simulink model "GA_fuzzy_sim"  (R2023a)
settings: Solver=VariableStepAuto  StartTime=0.0  StopTime=5  RelTol=1e-3
InitFcn:
  | m0=0.8; m1=0.5; m2=0.3; L1=0.3; L2=0.2; l1=0.15; l2=0.1; I1=0.015; I2=0.004; g=9.8;
  | d1=(m0+m1+m2);
  | d2=(m1*l1+m2*L1);
  | d3=m1*l1^2+m2*L1^2+I1;
  | d4=m2*l2;
  | d5=m2*L1*l2;
  | d6=m2*l2^2+I2;
libraries: fuzblock x1
settings Model: Creator=luand  LastModifiedBy=luand
settings DataIOCC: ReturnWorkspaceOutputs=off

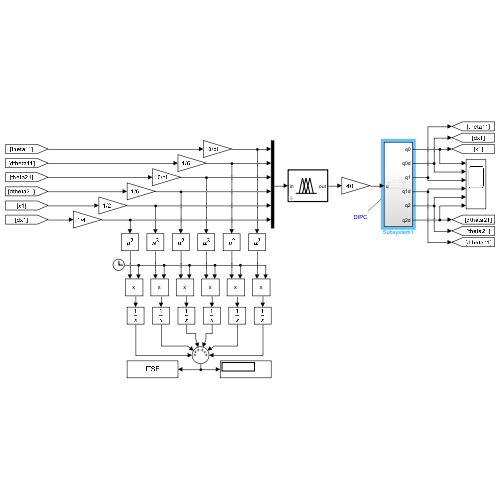
[thumbnail: Simulink's stored preview of the top-level diagram]
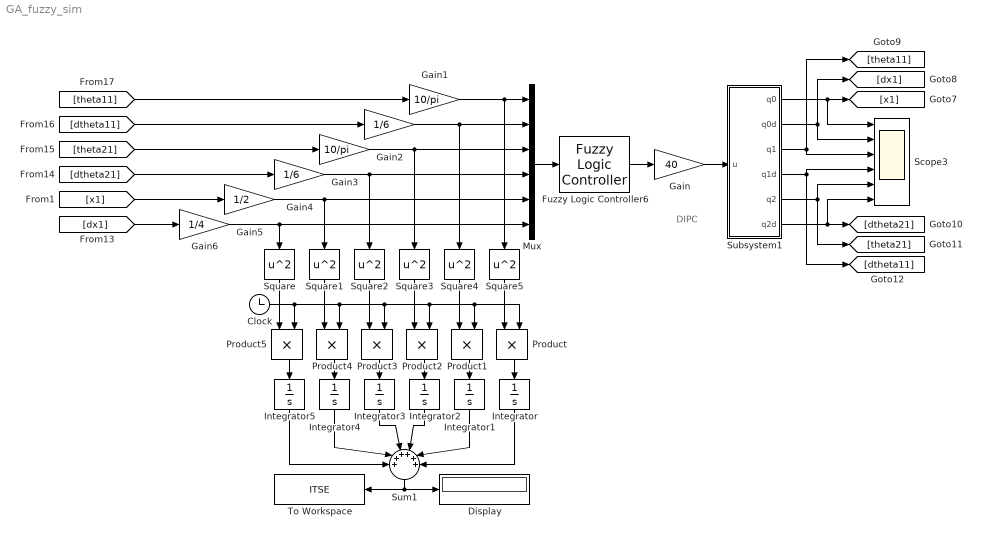
== system GA_fuzzy_sim ==
  note: DIPC
  Clock : Clock
  Display : Display
  Fuzzy Logic Controller6 : fuzblock/Fuzzy Logic  Controller  FIS='GAfis.fis'  OutputSampleNumber=101  DataType=double  FuzzifiedInputs=off  RuleFiringStrengths=off  RuleOutputs=off  AggregatedOutputs=off  SimulateUsing=Interpreted execution  OutOfRangeInputValueMessage=warning  NoRuleFiredMessage=warning  EmptyOutputFuzzySetMessage=warning
  Gain : Gain  Gain=40
  Gain1 : Gain  Gain=10/pi
  Gain2 : Gain  Gain=1/6
  Gain3 : Gain  Gain=10/pi
  Gain4 : Gain  Gain=1/6
  Gain5 : Gain  Gain=1/2
  Gain6 : Gain  Gain=1/4
  Integrator{,1..5} (6 alike) : Integrator
  Mux : Mux  Inputs=6
  Product{,1..5} (6 alike) : Product
  Scope3 : Scope  NumInputPorts=6
  Square{,1..5} (6 alike) : Math  Operator=square
  Subsystem1 : Subsystem
  Sum1 : Sum  Inputs=++++++
  To Workspace : ToWorkspace  VariableName=ITSE  SampleTime=-1
  wires:
  Square5/1 -> Product/1
  Subsystem1/5(q2) -> Scope3/5, [theta21]
  Square3/1 -> Product2/1
  Square2/1 -> Product3/1
  Square4/1 -> Product1/1
  [dtheta21] -> Gain4/1
  Product2/1 -> Integrator2/1
  [theta21] -> Gain3/1
  Clock/1 -> Product/2, Product1/2, Product2/2, Product3/2, Product4/2, Product5/2
  [dtheta11] -> Gain2/1
  Integrator4/1 -> Sum1/2
  Square1/1 -> Product4/1
  Subsystem1/6(q2d) -> [dtheta21], Scope3/6
  [theta11] -> Gain1/1
  Square/1 -> Product5/1
  Integrator2/1 -> Sum1/4
  Integrator3/1 -> Sum1/3
  Integrator/1 -> Sum1/6
  Product4/1 -> Integrator4/1
  Product/1 -> Integrator/1
  Mux/1 -> Fuzzy Logic Controller6/1
  Subsystem1/4(q1d) -> Scope3/4, [dtheta11]
  Integrator5/1 -> Sum1/1
  Sum1/1 -> Display/1, To Workspace/1
  [dx1] -> Gain6/1
  Product1/1 -> Integrator1/1
  Integrator1/1 -> Sum1/5
  Subsystem1/3(q1) -> Scope3/3, [theta11]
  Subsystem1/2(q0d) -> Scope3/2, [dx1]
  Product5/1 -> Integrator5/1
  Fuzzy Logic Controller6/1 -> Gain/1
  Product3/1 -> Integrator3/1
  Gain/1 -> Subsystem1/1(u)
  Subsystem1/1(q0) -> Scope3/1, [x1]
  [x1] -> Gain5/1
  Gain1/1 -> Square5/1, Mux/1
  Gain2/1 -> Square4/1, Mux/2
  Gain3/1 -> Square3/1, Mux/3
  Gain4/1 -> Square2/1, Mux/4
  Gain5/1 -> Square1/1, Mux/5
  Gain6/1 -> Square/1, Mux/6

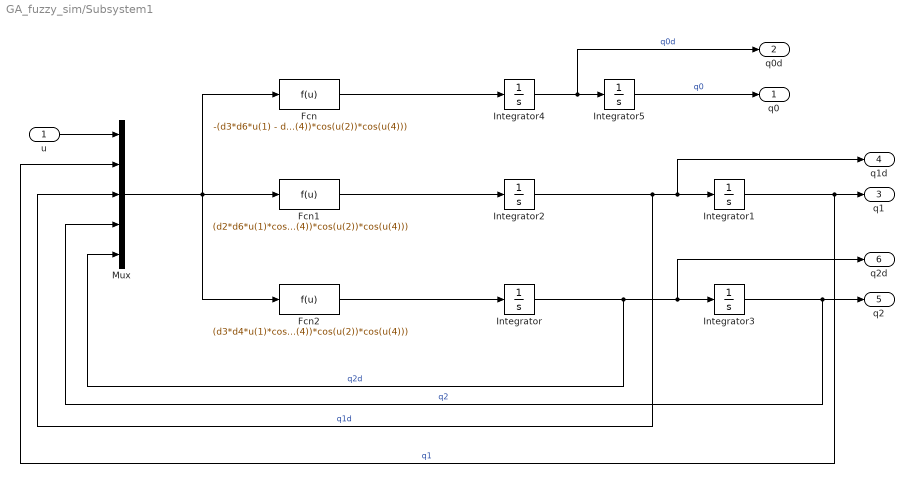
== system GA_fuzzy_sim/Subsystem1 ==
  u : Inport
  Fcn : Fcn  Expr=-(d3*d6*u(1) - d5^2*u(1)*cos(u(2) - u(4))^2 + d2*d3*d6*u(3)^2*sin(u(2)) + d3*d4*d6*u(5)^2*sin(u(4)) - d2*d5^2*u(3)^2*cos(u(2) - u(4))^2*sin(u(2)) - d4*d5^2*u(5)^2*cos(u(2) - u(4))^2*sin(u(4)) - d2^2*d6*g*cos(u(2))*sin(u(2)) - d3*d4^2*g*cos(u(4))*sin(u(4)) + d2*d5^2*u(3)^2*cos(u(2) - u(4))*sin(u(2) - u(4))*cos(u(2)) - d4*d5^2*u(5)^2*cos(u(2) - u(4))*sin(u(2) - u(4))*cos(u(4)) - d3*d4*d5*u(3)^2*sin(u(2) - u(4))*cos(u(4)) + d2*d5*d6*u(5)^2*sin(u(2) - u(4))*cos(u(2)) + d2*d4*d5*g*cos(u(2) - u(4))*cos(u(2))*sin(u(4)) + d2*d4*d5*g*cos(u(2) - u(4))*cos(u(4))*sin(u(2)))/(d3*d4^2*cos(u(4))^2 - d1*d3*d6 + d2^2*d6*cos(u(2))^2 + d1*d5^2*cos(u(2) - u(4))^2 - 2*d2*d4*d5*cos(u(2) - u(4))*cos(u(2))*cos(u(4)))
  Fcn1 : Fcn  Expr=(d2*d6*u(1)*cos(u(2)) + d2*d4^2*g*cos(u(4))^2*sin(u(2)) + d2^2*d6*u(3)^2*cos(u(2))*sin(u(2)) + d1*d5^2*u(3)^2*cos(u(2) - u(4))*sin(u(2) - u(4)) + d1*d5*d6*u(5)^2*sin(u(2) - u(4)) - d4*d5*u(1)*cos(u(2) - u(4))*cos(u(4)) - d4^2*d5*u(5)^2*sin(u(2) - u(4))*cos(u(4))^2 - d1*d2*d6*g*sin(u(2)) - d4^2*d5*u(5)^2*cos(u(2) - u(4))*cos(u(4))*sin(u(4)) + d2*d4*d6*u(5)^2*cos(u(2))*sin(u(4)) - d2*d4^2*g*cos(u(2))*cos(u(4))*sin(u(4)) + d1*d4*d5*g*cos(u(2) - u(4))*sin(u(4)) - d2*d4*d5*u(3)^2*cos(u(2) - u(4))*cos(u(4))*sin(u(2)) - d2*d4*d5*u(3)^2*sin(u(2) - u(4))*cos(u(2))*cos(u(4)))/(d3*d4^2*cos(u(4))^2 - d1*d3*d6 + d2^2*d6*cos(u(2))^2 + d1*d5^2*cos(u(2) - u(4))^2 - 2*d2*d4*d5*cos(u(2) - u(4))*cos(u(2))*cos(u(4)))
  Fcn2 : Fcn  Expr=(d3*d4*u(1)*cos(u(4)) + d2^2*d4*g*cos(u(2))^2*sin(u(4)) + d3*d4^2*u(5)^2*cos(u(4))*sin(u(4)) - d1*d5^2*u(5)^2*cos(u(2) - u(4))*sin(u(2) - u(4)) - d1*d3*d5*u(3)^2*sin(u(2) - u(4)) - d2*d5*u(1)*cos(u(2) - u(4))*cos(u(2)) + d2^2*d5*u(3)^2*sin(u(2) - u(4))*cos(u(2))^2 - d1*d3*d4*g*sin(u(4)) - d2^2*d5*u(3)^2*cos(u(2) - u(4))*cos(u(2))*sin(u(2)) + d2*d3*d4*u(3)^2*cos(u(4))*sin(u(2)) - d2^2*d4*g*cos(u(2))*cos(u(4))*sin(u(2)) + d1*d2*d5*g*cos(u(2) - u(4))*sin(u(2)) - d2*d4*d5*u(5)^2*cos(u(2) - u(4))*cos(u(2))*sin(u(4)) + d2*d4*d5*u(5)^2*sin(u(2) - u(4))*cos(u(2))*cos(u(4)))/(d3*d4^2*cos(u(4))^2 - d1*d3*d6 + d2^2*d6*cos(u(2))^2 + d1*d5^2*cos(u(2) - u(4))^2 - 2*d2*d4*d5*cos(u(2) - u(4))*cos(u(2))*cos(u(4)))
  Integrator : Integrator  LimitOutput=on  UpperSaturationLimit=10  LowerSaturationLimit=-10
  Integrator1 : Integrator  InitialCondition=pi/10  LimitOutput=on  UpperSaturationLimit=10  LowerSaturationLimit=-10
  Integrator2 : Integrator  LimitOutput=on  UpperSaturationLimit=10  LowerSaturationLimit=-10
  Integrator3 : Integrator  InitialCondition=pi/10  LimitOutput=on  UpperSaturationLimit=10  LowerSaturationLimit=-10
  Integrator4 : Integrator  LimitOutput=on  UpperSaturationLimit=50  LowerSaturationLimit=-50
  Integrator5 : Integrator  LimitOutput=on  UpperSaturationLimit=50  LowerSaturationLimit=-50
  Mux : Mux  Inputs=5
  q0 : Outport  VectorParamsAs1DForOutWhenUnconnected=off
  q0d : Outport  Port=2  VectorParamsAs1DForOutWhenUnconnected=off
  q1 : Outport  Port=3  VectorParamsAs1DForOutWhenUnconnected=off
  q1d : Outport  Port=4  VectorParamsAs1DForOutWhenUnconnected=off
  q2 : Outport  Port=5  VectorParamsAs1DForOutWhenUnconnected=off
  q2d : Outport  Port=6  VectorParamsAs1DForOutWhenUnconnected=off
  wires:
  Integrator/1 -> Mux/5, q2d/1, Integrator3/1  "q2d"
  u/1 -> Mux/1
  Integrator1/1 -> Mux/2, q1/1  "q1"
  Integrator4/1 -> q0d/1, Integrator5/1  "q0d"
  Integrator5/1 -> q0/1  "q0"
  Integrator2/1 -> Mux/3, q1d/1, Integrator1/1  "q1d"
  Integrator3/1 -> Mux/4, q2/1  "q2"
  Mux/1 -> Fcn2/1, Fcn/1, Fcn1/1
  Fcn/1 -> Integrator4/1
  Fcn1/1 -> Integrator2/1
  Fcn2/1 -> Integrator/1
